simulink model "speed_modelo_definitivo"  (R2022b)
settings: Solver=VariableStepAuto  StartTime=0.0  StopTime=6  FixedStep=0.01  MaxStep=0.00005  RelTol=1e-3
undefined symbols (not defined in the file or in its folder): airgap_drag, corriente_inductancia, Force_drag, frecuencia, frecuencia_freno, FuerzaX_acel, FuerzaX_freno, FuerzaY_acel, Ipeak, mass, p1, p2, pole_length, r, slip, valores_inductancia, VDC, vel_drag, vel_motor_freno
libraries: slpidlib x2
settings Model: Creator=mique  LastModifiedBy=mique
settings SolverCC: ZeroCrossAlgorithm=Adaptive
settings DebuggingCC: IgnoredZcDiagnostic=none

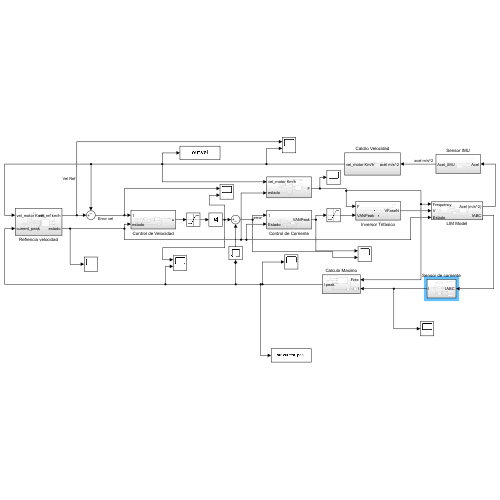
[thumbnail: Simulink's stored preview of the top-level diagram]
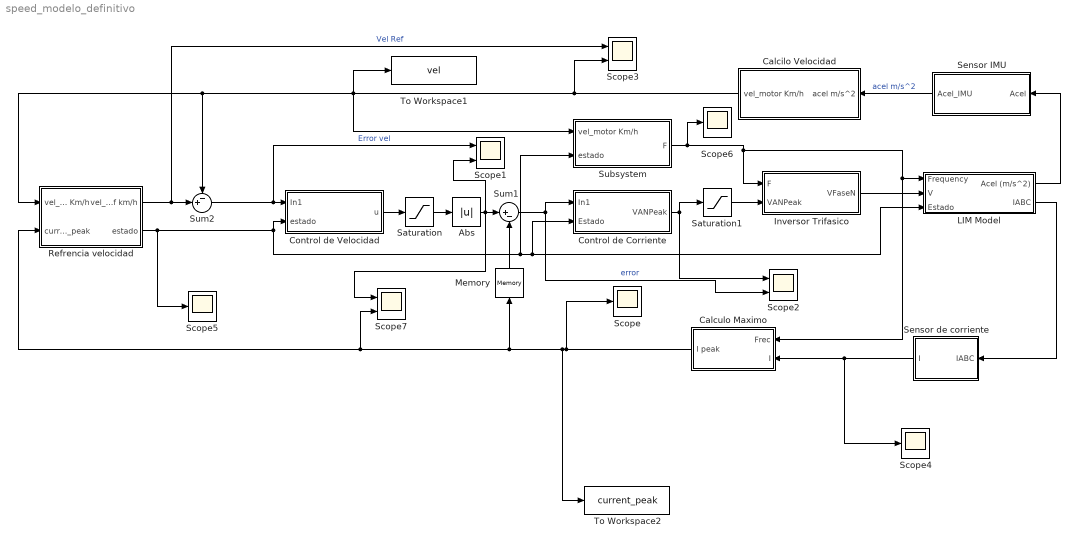
== system speed_modelo_definitivo ==
  Abs : Abs  SaturateOnIntegerOverflow=off
  Calcilo Velocidad : Subsystem
  Calculo Maximo : Subsystem
  Control de Corriente : Subsystem
  Control de Velocidad : Subsystem
  Inversor Trifasico : Subsystem
  LIM Model : Subsystem
  Memory : Memory
  Refrencia velocidad : Subsystem
  Saturation : Saturate  UpperLimit=100  LowerLimit=-100
  Saturation1 : Saturate  UpperLimit=200/sqrt(3)  LowerLimit=0
  Scope{,4..6} (4 alike) : Scope
  Scope{1..3,7} (4 alike) : Scope  NumInputPorts=2
  Sensor IMU : Subsystem
  Sensor de corriente : Subsystem
  Subsystem : Subsystem
  Sum1 : Sum  Inputs=|+-
  Sum2 : Sum  Inputs=-+|
  To Workspace1 : ToWorkspace  VariableName=vel  SampleTime=-1
  To Workspace2 : ToWorkspace  VariableName=current_peak  SaveFormat=Timeseries  SampleTime=-1
  wires:
  LIM Model/1(Acel (m/s^2)) -> Sensor IMU/1(Acel)
  Sum1/1 -> Control de Corriente/1(In1), Scope2/2  "error"
  Refrencia velocidad/1(vel_ref km/h) -> Scope3/1, Sum2/2  "Vel Ref"
  Control de Velocidad/1(u) -> Saturation/1
  Inversor Trifasico/1(VFaseN) -> LIM Model/2("V ")
  Memory/1 -> Sum1/2
  Sensor de corriente/1(I) -> Scope4/1, Calculo Maximo/2(I)
  Control de Corriente/1(VANPeak) -> Saturation1/1, Scope2/1
  Saturation1/1 -> Inversor Trifasico/2(VANPeak)
  Subsystem/1(F) -> Scope6/1, Calculo Maximo/1(Frec), LIM Model/1(Frequency), Inversor Trifasico/1(F)
  Calculo Maximo/1(I peak) -> To Workspace2/1, Scope7/2, Refrencia velocidad/2(current_peak), Memory/1, Scope/1
  LIM Model/2(IABC) -> Sensor de corriente/1(IABC)
  Calcilo Velocidad/1(vel_motor Km/h) -> Scope3/2, Refrencia velocidad/1(vel_motor Km/h), Sum2/1, To Workspace1/1, Subsystem/1(vel_motor Km/h)
  Sensor IMU/1(Acel_IMU) -> Calcilo Velocidad/1(acel m/s^2)  "acel m/s^2"
  Sum2/1 -> Scope1/1, Control de Velocidad/1(In1)  "Error vel"
  Refrencia velocidad/2(estado) -> Scope5/1, Control de Velocidad/2(estado), LIM Model/3(Estado), Control de Corriente/2(Estado), Subsystem/2(estado)
  Saturation/1 -> Abs/1
  Abs/1 -> Scope7/1, Sum1/1, Scope1/2

== system speed_modelo_definitivo/Calcilo Velocidad ==
  acel m/s^2 : Inport
  Gain : Gain  Gain=3.6
  Integrator1 : Integrator
  vel_motor Km/h : Outport
  wires:
  Gain/1 -> vel_motor Km/h/1  "vel_motor Km/h"
  Integrator1/1 -> Gain/1  "vel_motor m/s"
  acel m/s^2/1 -> Integrator1/1

== system speed_modelo_definitivo/Calculo Maximo ==
  Frec : Inport
  I : Inport  Port=2
  Abs : Abs  SaturateOnIntegerOverflow=off
  Clock : Clock
  MATLAB Function : MATLAB Function  TreatAsAtomicUnit=on
  Scope : Scope  NumInputPorts=2
  I peak : Outport
  wires:
  Frec/1 -> MATLAB Function/1(frecuencia)
  I/1 -> MATLAB Function/2(valores), Abs/1
  MATLAB Function/1(maximo) -> I peak/1, Scope/1
  Clock/1 -> MATLAB Function/3(tiempo)
  Abs/1 -> Scope/2

== system speed_modelo_definitivo/Control de Corriente ==
  note: Parametros obtenidos con el PID tuner
  In1 : Inport
  Estado : Inport  Port=2
  Discrete PID Controller1 : slpidlib/PID Controller  Controller=PI  Form=Parallel  TimeDomain=Discrete-time  UseExternalTs=off  SampleTime=0.0002  IntegratorMethod=Forward Euler  FilterMethod=Forward Euler  ControllerParametersSource=internal  P=1  I=25  UseKiTs=off  D=0.3  N=2  UseFilter=on  TunerSelectOption=Transfer Function Based (PID Tuner App)  InitialConditionSource=internal  InitialConditionForIntegrator=0  InitialConditionForFilter=0  DifferentiatorICPrevScaledInput=0  ExternalReset=level  TrackingMode=off  Kt=1  LimitOutput=off  SatLimitsSource=internal  UpperSaturationLimit=VDC/sqrt(3)  LowerSaturationLimit=-VDC/sqrt(3)  LinearizeAsGain=off  AntiWindupMode=back-calculation  Kb=20  LimitIntegrator=off  UpperIntegratorSaturationLimit=15  LowerIntegratorSaturationLimit=-15  POutMin=[]  POutMax=[]  IOutMin=[]  IOutMax=[]  DOutMin=[]  DOutMax=[]  NOutMin=[]  NOutMax=[]  SumOutMin=[]  SumOutMax=[]  SaturationOutMin=[]  SaturationOutMax=[]  PParamMin=[]  PParamMax=[]  IParamMin=[]  IParamMax=[]  DParamMin=[]  DParamMax=[]  NParamMin=[]  NParamMax=[]  KbParamMin=[]  KbParamMax=[]  KtParamMin=[]  KtParamMax=[]  KbOutMin=[]  KbOutMax=[]  KtOutMin=[]  KtOutMax=[]  IntegratorOutMin=[]  IntegratorOutMax=[]  FilterOutMin=[]  FilterOutMax=[]  SumI1OutMin=[]  SumI1OutMax=[]  SumI2OutMin=[]  SumI2OutMax=[]  SumI3OutMin=[]  SumI3OutMax=[]  SumI4OutMin=[]  SumI4OutMax=[]  SumDOutMin=[]  SumDOutMax=[]  DifferentiatorOutMin=[]  DifferentiatorOutMax=[]  FilterDiffOutCoefMin=[]  FilterDiffOutCoefMax=[]  ReciprocalOutMin=[]  ReciprocalOutMax=[]  SumDenOutMin=[]  SumDenOutMax=[]  SumNumOutMin=[]  SumNumOutMax=[]  DivideOutMin=[]  DivideOutMax=[]  UdiffTsProdOutMin=[]  UdiffTsProdOutMax=[]  NTsProdOutMin=[]  NTsProdOutMax=[]  UintegralTsProdOutMin=[]  UintegralTsProdOutMax=[]  UngainTsProdOutMin=[]  UngainTsProdOutMax=[]  ClampingZeroOutDataTypeStr=Inherit: Inherit via back propagation  ClampingZeroOutMin=[]  ClampingZeroOutMax=[]  FilterDenConstantOutDataTypeStr=Inherit: Inherit via back propagation  FilterDenConstantOutMin=[]  FilterDenConstantOutMax=[]  PCopyOutDataTypeStr=Inherit: Inherit via back propagation  PCopyOutMin=[]  PCopyOutMax=[]  NCopyOutDataTypeStr=Inherit: Inherit via back propagation  NCopyOutMin=[]  NCopyOutMax=[]  IntegratorContinuousStateAttributes=''  IntegratorStateMustResolveToSignalObject=off  IntegratorRTWStateStorageClass=Auto  FilterContinuousStateAttributes=''  FilterStateMustResolveToSignalObject=off  FilterRTWStateStorageClass=Auto  ParallelPVariant=InternalParameters  IdealPVariant=Disabled  IVariant=InternalParameters  DVariant=Disabled  IntegratorVariant=Discrete  SatVariant=Disabled  AWVariant=Passthrough  PCopyVariant=Disabled  TRVariant=Disabled  FdbkBlocksVariant=Forward  IdealPFdbkVariant=Disabled  SatFdbkVariant=Disabled  DerivativeFilterVariant=Disabled  NVariant=Disabled  NCopyVariant=Disabled_SignalSpec  FilterICVariant=Disabled  IntegratorICVariant=InternalICs  ExternalResetVariant=ExternalReset  TRSumVariant=Passthrough  SumFdbkVariant=Disabled  SumVariant=Sum_PI  TsampFilterVariant=InternalTs  TsampNgainVariant=Passthrough  TsampIntegralVariant=Passthrough  ExternalSaturationOutDataTypeStr=Inherit: Same as second input
      settings: LibrarySourceBlock=simulink/Discrete/Discrete PID Controller
  MATLAB Function : MATLAB Function  TreatAsAtomicUnit=on
  Memory : Memory
  VANPeak : Outport
  wires:
  In1/1 -> Discrete PID Controller1/1
  Discrete PID Controller1/1 -> MATLAB Function/1(u)
  Estado/1 -> MATLAB Function/2(estado)
  MATLAB Function/1(y) -> VANPeak/1
  MATLAB Function/2(reset) -> Memory/1
  Memory/1 -> Discrete PID Controller1/2

== system speed_modelo_definitivo/Control de Velocidad ==
  note: Parametros obtenidos con el PID tuner
  In1 : Inport
  estado : Inport  Port=2
  Discrete PID Controller1 : slpidlib/PID Controller  Controller=PI  Form=Parallel  TimeDomain=Discrete-time  UseExternalTs=off  SampleTime=0.001  IntegratorMethod=Forward Euler  FilterMethod=Forward Euler  ControllerParametersSource=internal  P=40  I=2  UseKiTs=off  D=0.2  N=10  UseFilter=on  TunerSelectOption=Transfer Function Based (PID Tuner App)  InitialConditionSource=internal  InitialConditionForIntegrator=0  InitialConditionForFilter=0  DifferentiatorICPrevScaledInput=0  ExternalReset=level  TrackingMode=off  Kt=1  LimitOutput=off  SatLimitsSource=internal  UpperSaturationLimit=100  LowerSaturationLimit=-100  LinearizeAsGain=off  AntiWindupMode=clamping  Kb=0.1  LimitIntegrator=off  UpperIntegratorSaturationLimit=15  LowerIntegratorSaturationLimit=-15  POutMin=[]  POutMax=[]  IOutMin=[]  IOutMax=[]  DOutMin=[]  DOutMax=[]  NOutMin=[]  NOutMax=[]  SumOutMin=[]  SumOutMax=[]  SaturationOutMin=[]  SaturationOutMax=[]  PParamMin=[]  PParamMax=[]  IParamMin=[]  IParamMax=[]  DParamMin=[]  DParamMax=[]  NParamMin=[]  NParamMax=[]  KbParamMin=[]  KbParamMax=[]  KtParamMin=[]  KtParamMax=[]  KbOutMin=[]  KbOutMax=[]  KtOutMin=[]  KtOutMax=[]  IntegratorOutMin=[]  IntegratorOutMax=[]  FilterOutMin=[]  FilterOutMax=[]  SumI1OutMin=[]  SumI1OutMax=[]  SumI2OutMin=[]  SumI2OutMax=[]  SumI3OutMin=[]  SumI3OutMax=[]  SumI4OutMin=[]  SumI4OutMax=[]  SumDOutMin=[]  SumDOutMax=[]  DifferentiatorOutMin=[]  DifferentiatorOutMax=[]  FilterDiffOutCoefMin=[]  FilterDiffOutCoefMax=[]  ReciprocalOutMin=[]  ReciprocalOutMax=[]  SumDenOutMin=[]  SumDenOutMax=[]  SumNumOutMin=[]  SumNumOutMax=[]  DivideOutMin=[]  DivideOutMax=[]  UdiffTsProdOutMin=[]  UdiffTsProdOutMax=[]  NTsProdOutMin=[]  NTsProdOutMax=[]  UintegralTsProdOutMin=[]  UintegralTsProdOutMax=[]  UngainTsProdOutMin=[]  UngainTsProdOutMax=[]  ClampingZeroOutDataTypeStr=Inherit: Inherit via back propagation  ClampingZeroOutMin=[]  ClampingZeroOutMax=[]  FilterDenConstantOutDataTypeStr=Inherit: Inherit via back propagation  FilterDenConstantOutMin=[]  FilterDenConstantOutMax=[]  PCopyOutDataTypeStr=Inherit: Inherit via back propagation  PCopyOutMin=[]  PCopyOutMax=[]  NCopyOutDataTypeStr=Inherit: Inherit via back propagation  NCopyOutMin=[]  NCopyOutMax=[]  IntegratorContinuousStateAttributes=''  IntegratorStateMustResolveToSignalObject=off  IntegratorRTWStateStorageClass=Auto  FilterContinuousStateAttributes=''  FilterStateMustResolveToSignalObject=off  FilterRTWStateStorageClass=Auto  ParallelPVariant=InternalParameters  IdealPVariant=Disabled  IVariant=InternalParameters  DVariant=Disabled  IntegratorVariant=Discrete  SatVariant=Disabled  AWVariant=Passthrough  PCopyVariant=Disabled  TRVariant=Disabled  FdbkBlocksVariant=Forward  IdealPFdbkVariant=Disabled  SatFdbkVariant=Disabled  DerivativeFilterVariant=Disabled  NVariant=Disabled  NCopyVariant=Disabled_SignalSpec  FilterICVariant=Disabled  IntegratorICVariant=InternalICs  ExternalResetVariant=ExternalReset  TRSumVariant=Passthrough  SumFdbkVariant=Disabled  SumVariant=Sum_PI  TsampFilterVariant=InternalTs  TsampNgainVariant=Passthrough  TsampIntegralVariant=Passthrough  ExternalSaturationOutDataTypeStr=Inherit: Same as second input
      settings: LibrarySourceBlock=simulink/Discrete/Discrete PID Controller
  MATLAB Function : MATLAB Function  TreatAsAtomicUnit=on
  Memory : Memory
  u : Outport
  wires:
  Discrete PID Controller1/1 -> MATLAB Function/1(i)
  In1/1 -> Discrete PID Controller1/1
  MATLAB Function/1(i_ref) -> u/1
  estado/1 -> MATLAB Function/2(estado)
  MATLAB Function/2(reset) -> Memory/1
  Memory/1 -> Discrete PID Controller1/2

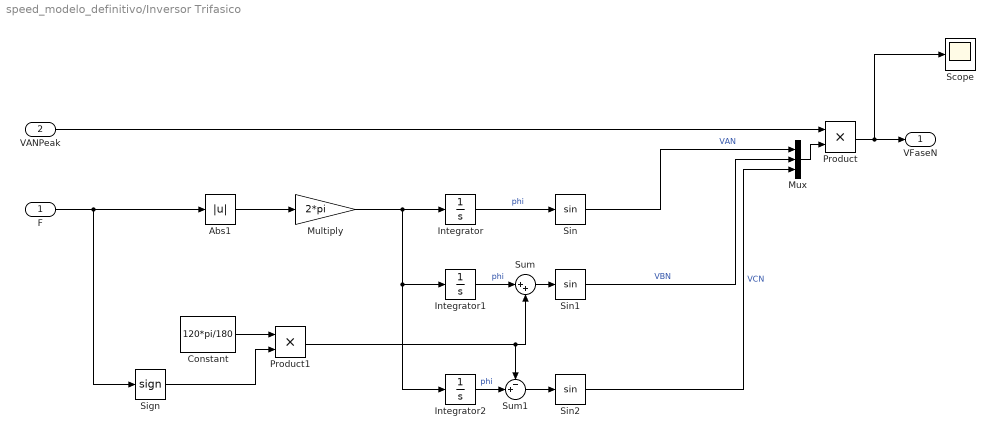
== system speed_modelo_definitivo/Inversor Trifasico ==
  F : Inport
  VANPeak : Inport  Port=2
  Abs1 : Abs  SaturateOnIntegerOverflow=off
  Constant : Constant  Value=120*pi/180
  Integrator : Integrator  WrapState=on  WrappedStateUpperValue=2*pi  WrappedStateLowerValue=0
  Integrator1 : Integrator  WrapState=on  WrappedStateUpperValue=2*pi  WrappedStateLowerValue=0
  Integrator2 : Integrator  WrapState=on  WrappedStateUpperValue=2*pi  WrappedStateLowerValue=0
  Multiply : Gain  Gain=2*pi
  Mux : Mux  Inputs=3
  Product : Product
  Product1 : Product
  Scope : Scope
  Sign : Signum
  Sin : Trigonometry
  Sin1 : Trigonometry
  Sin2 : Trigonometry
  Sum : Sum  Inputs=|++
  Sum1 : Sum  Inputs=-+|
  VFaseN : Outport
  wires:
  Integrator/1 -> Sin/1  "phi"
  Multiply/1 -> Integrator2/1, Integrator1/1, Integrator/1
  VANPeak/1 -> Product/1
  Sin/1 -> Mux/1  "VAN"
  Sin1/1 -> Mux/2  "VBN"
  Sin2/1 -> Mux/3  "VCN"
  Integrator1/1 -> Sum/1  "phi"
  Sum/1 -> Sin1/1
  Sum1/1 -> Sin2/1
  Integrator2/1 -> Sum1/2  "phi"
  Mux/1 -> Product/2
  Product/1 -> Scope/1, VFaseN/1
  F/1 -> Sign/1, Abs1/1
  Abs1/1 -> Multiply/1
  Constant/1 -> Product1/1
  Sign/1 -> Product1/2
  Product1/1 -> Sum1/1, Sum/2

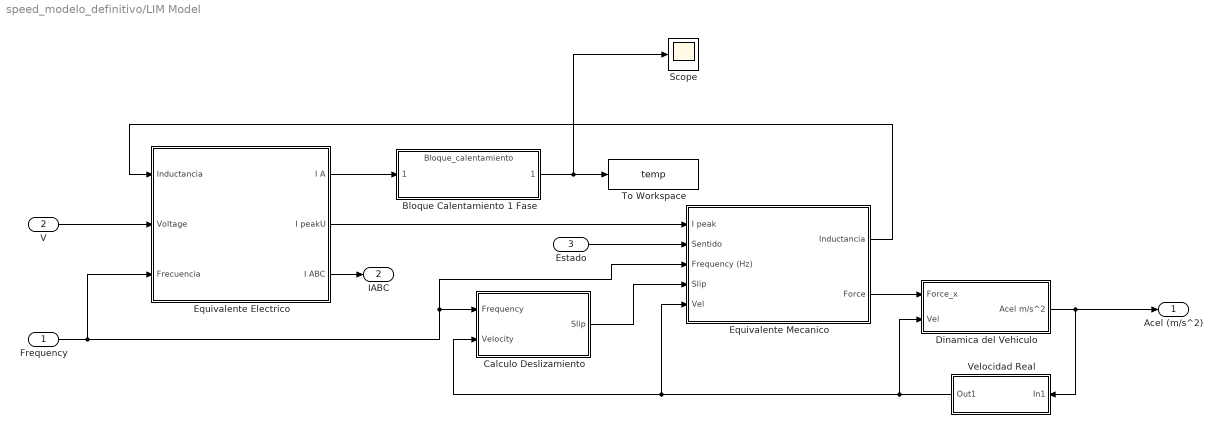
== system speed_modelo_definitivo/LIM Model ==
  Frequency : Inport
  "V " : Inport  Port=2
  Estado : Inport  Port=3
  Bloque Calentamiento 1 Fase : ModelReference  ModelNameDialog=Bloque_calentamiento.slx  SimulationMode=Normal  ModelReferenceVersion=3.9
  Calculo Deslizamiento : Subsystem
  Dinamica del Vehiculo : Subsystem
  Equivalente Electrico : Subsystem
  Equivalente Mecanico : Subsystem
  Scope : Scope
  To Workspace : ToWorkspace  VariableName=temp  SaveFormat=Timeseries  SampleTime=-1
  Velocidad Real : Subsystem
  Acel (m/s^2) : Outport
  IABC : Outport  Port=2
  wires:
  Dinamica del Vehiculo/1(Acel m/s^2) -> Acel (m/s^2)/1, Velocidad Real/1(In1)
  Equivalente Electrico/2(I peakU) -> Equivalente Mecanico/1(I peak)
  Frequency/1 -> Equivalente Electrico/3(Frecuencia), Equivalente Mecanico/3(Frequency (Hz)), Calculo Deslizamiento/1(Frequency)
  "V "/1 -> Equivalente Electrico/2(Voltage)
  Equivalente Electrico/1(I A) -> Bloque Calentamiento 1 Fase/1
  Estado/1 -> Equivalente Mecanico/2(Sentido)
  Calculo Deslizamiento/1(Slip) -> Equivalente Mecanico/4(Slip)
  Equivalente Mecanico/2(Force) -> Dinamica del Vehiculo/1(Force_x)
  Equivalente Electrico/3(I ABC) -> IABC/1
  Velocidad Real/1(Out1) -> Dinamica del Vehiculo/2(Vel), Calculo Deslizamiento/2(Velocity), Equivalente Mecanico/5(Vel)
  Bloque Calentamiento 1 Fase/1 -> Scope/1, To Workspace/1
  Equivalente Mecanico/1(Inductancia) -> Equivalente Electrico/1(Inductancia)

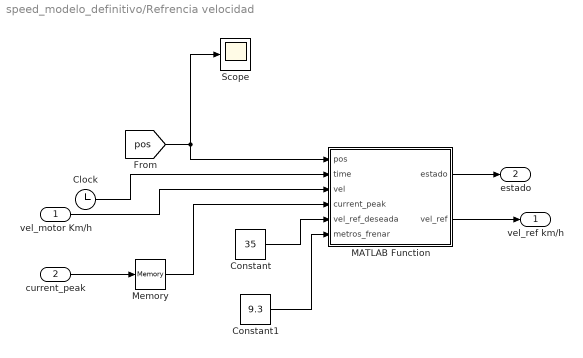
== system speed_modelo_definitivo/Refrencia velocidad ==
  vel_motor Km/h : Inport
  current_peak : Inport  Port=2
  Clock : Clock
  Constant : Constant  Value=35
  Constant1 : Constant  Value=9.3
  MATLAB Function : MATLAB Function  TreatAsAtomicUnit=on
  Memory : Memory
  Scope : Scope
  vel_ref km/h : Outport
  estado : Outport  Port=2
  wires:
  MATLAB Function/2(vel_ref) -> vel_ref km/h/1
  vel_motor Km/h/1 -> MATLAB Function/3(vel)
  Clock/1 -> MATLAB Function/2(time)
  [pos] -> MATLAB Function/1(pos), Scope/1
  current_peak/1 -> Memory/1
  Memory/1 -> MATLAB Function/4(current_peak)
  MATLAB Function/1(estado) -> estado/1
  Constant/1 -> MATLAB Function/5(vel_ref_deseada)
  Constant1/1 -> MATLAB Function/6(metros_frenar)

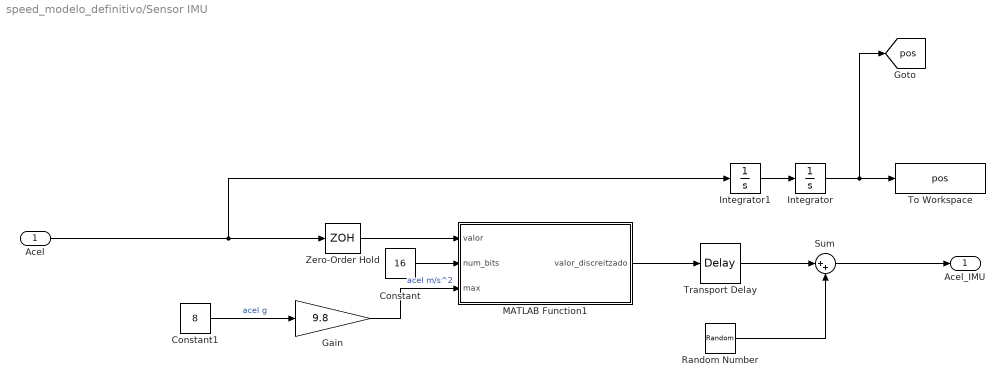
== system speed_modelo_definitivo/Sensor IMU ==
  Acel : Inport
  Constant : Constant  Value=16
  Constant1 : Constant  Value=8
  Gain : Gain  Gain=9.8
  Integrator : Integrator
  Integrator1 : Integrator
  MATLAB Function1 : MATLAB Function  TreatAsAtomicUnit=on
  Random Number : RandomNumber  Variance=0.1  SampleTime=0.001
  Sum : Sum  Inputs=|++
  To Workspace : ToWorkspace  VariableName=pos  SampleTime=-1
  Transport Delay : TransportDelay  DelayTime=0.001
  Zero-Order Hold : ZeroOrderHold  SampleTime=0.001
  Acel_IMU : Outport
  tag scope: pos=global
  wires:
  MATLAB Function1/1(valor_discreitzado) -> Transport Delay/1
  Zero-Order Hold/1 -> MATLAB Function1/1(valor)
  Constant1/1 -> Gain/1  "acel g"
  Constant/1 -> MATLAB Function1/2(num_bits)
  Gain/1 -> MATLAB Function1/3(max)  "acel m/s^2"
  Transport Delay/1 -> Sum/1
  Acel/1 -> Integrator1/1, Zero-Order Hold/1
  Sum/1 -> Acel_IMU/1
  Random Number/1 -> Sum/2
  Integrator/1 -> [pos], To Workspace/1
  Integrator1/1 -> Integrator/1

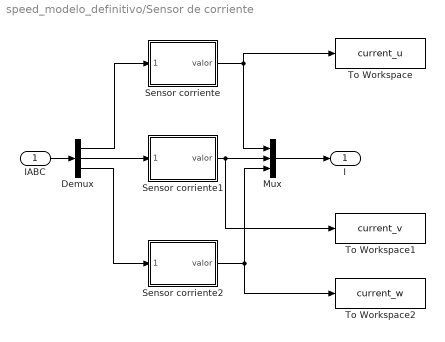
== system speed_modelo_definitivo/Sensor de corriente ==
  IABC : Inport
  Demux : Demux  Outputs=3
  Mux : Mux  Inputs=3
  Sensor corriente : Subsystem
  Sensor corriente1 : Subsystem
  Sensor corriente2 : Subsystem
  To Workspace : ToWorkspace  VariableName=current_u  SaveFormat=Timeseries  SampleTime=-1
  To Workspace1 : ToWorkspace  VariableName=current_v  SaveFormat=Timeseries  SampleTime=-1
  To Workspace2 : ToWorkspace  VariableName=current_w  SaveFormat=Timeseries  SampleTime=-1
  I : Outport
  wires:
  IABC/1 -> Demux/1
  Demux/2 -> Sensor corriente1/1(Current)
  Demux/1 -> Sensor corriente/1(Current)
  Demux/3 -> Sensor corriente2/1(Current)
  Sensor corriente1/1(valor) -> To Workspace1/1, Mux/2
  Mux/1 -> I/1
  Sensor corriente2/1(valor) -> Mux/3, To Workspace2/1
  Sensor corriente/1(valor) -> To Workspace/1, Mux/1

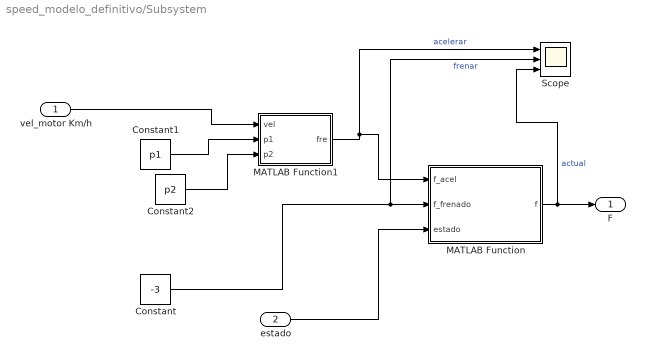
== system speed_modelo_definitivo/Subsystem ==
  vel_motor Km/h : Inport
  estado : Inport  Port=2
  Constant : Constant  Value=-3
  Constant1 : Constant  Value=p1
  Constant2 : Constant  Value=p2
  MATLAB Function : MATLAB Function  TreatAsAtomicUnit=on
  MATLAB Function1 : MATLAB Function  TreatAsAtomicUnit=on
  Scope : Scope  NumInputPorts=3
  F : Outport
  wires:
  vel_motor Km/h/1 -> MATLAB Function1/1(vel)
  estado/1 -> MATLAB Function/3(estado)
  MATLAB Function1/1(fre) -> Scope/1, MATLAB Function/1(f_acel)  "acelerar"
  MATLAB Function/1(f) -> Scope/3, F/1  "actual"
  Constant1/1 -> MATLAB Function1/2(p1)
  Constant2/1 -> MATLAB Function1/3(p2)
  Constant/1 -> Scope/2, MATLAB Function/2(f_frenado)  "frenar"

== system speed_modelo_definitivo/LIM Model/Calculo Deslizamiento ==
  Frequency : Inport
  Velocity : Inport  Port=2
  Constant : Constant  Value=pole_length
  Divide : Product  Inputs=**
  Gain : Gain  Gain=7.2
  MATLAB Function : MATLAB Function  TreatAsAtomicUnit=on
  Slip : Outport
  wires:
  Frequency/1 -> Gain/1
  MATLAB Function/1(slip) -> Slip/1
  Gain/1 -> Divide/2
  Constant/1 -> Divide/1
  Divide/1 -> MATLAB Function/1(we)
  Velocity/1 -> MATLAB Function/2(wm)

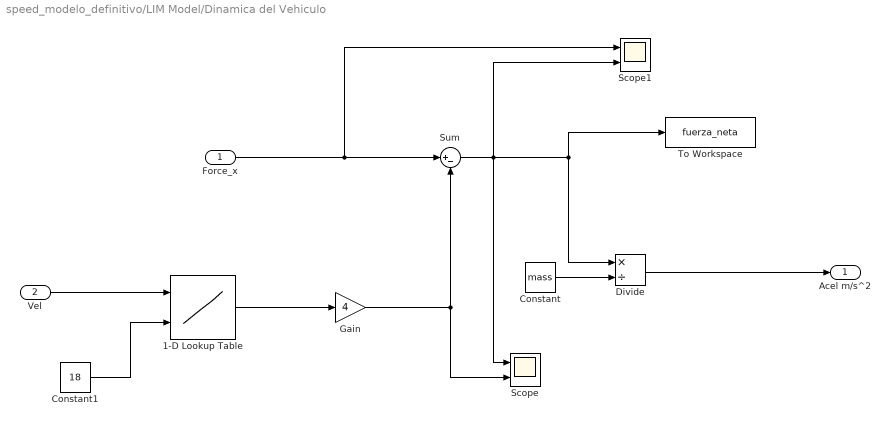
== system speed_modelo_definitivo/LIM Model/Dinamica del Vehiculo ==
  Force_x : Inport
  Vel : Inport  Port=2
  1-D Lookup Table : Lookup_n-D  BreakpointsForDimension1=vel_drag  BreakpointsForDimension2=airgap_drag  Table=Force_drag  InternalRulePriority=Speed  RndMeth=Simplest
      settings: InputPortMap=u0,u1
  Constant : Constant  Value=mass
  Constant1 : Constant  Value=18
  Divide : Product  Inputs=*/
  Gain : Gain  Gain=4
  Scope : Scope  NumInputPorts=2
  Scope1 : Scope  NumInputPorts=2
  Sum : Sum  Inputs=|+-
  To Workspace : ToWorkspace  VariableName=fuerza_neta  SampleTime=-1
  Acel m/s^2 : Outport
  wires:
  Divide/1 -> Acel m/s^2/1
  Constant/1 -> Divide/2
  Force_x/1 -> Sum/1, Scope1/1
  Sum/1 -> To Workspace/1, Divide/1, Scope1/2, Scope/1
  Constant1/1 -> 1-D Lookup Table/2
  1-D Lookup Table/1 -> Gain/1
  Gain/1 -> Scope/2, Sum/2
  Vel/1 -> 1-D Lookup Table/1

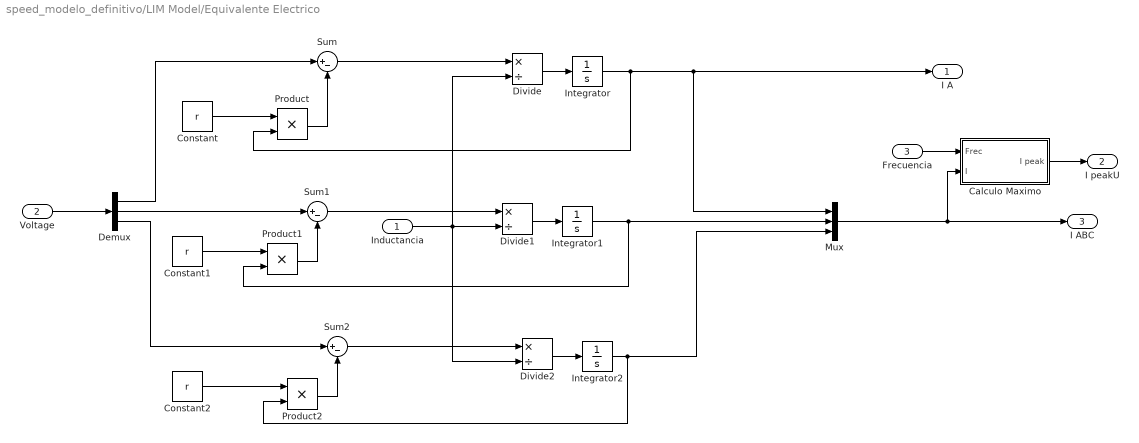
== system speed_modelo_definitivo/LIM Model/Equivalente Electrico ==
  Inductancia : Inport
  Voltage : Inport  Port=2
  Frecuencia : Inport  Port=3
  Calculo Maximo : Subsystem
  Constant : Constant  Value=r
  Constant1 : Constant  Value=r
  Constant2 : Constant  Value=r
  Demux : Demux  Outputs=3
  Divide : Product  Inputs=*/
  Divide1 : Product  Inputs=*/
  Divide2 : Product  Inputs=*/
  Integrator : Integrator
  Integrator1 : Integrator
  Integrator2 : Integrator
  Mux : Mux  Inputs=3
  Product : Product
  Product1 : Product
  Product2 : Product
  Sum : Sum  Inputs=|+-
  Sum1 : Sum  Inputs=|+-
  Sum2 : Sum  Inputs=|+-
  I A : Outport
  I peakU : Outport  Port=2
  I ABC : Outport  Port=3
  wires:
  Integrator/1 -> I A/1, Mux/1, Product/2
  Constant/1 -> Product/1
  Product/1 -> Sum/2
  Divide/1 -> Integrator/1
  Sum/1 -> Divide/1
  Sum1/1 -> Divide1/1
  Product1/1 -> Sum1/2
  Divide1/1 -> Integrator1/1
  Integrator1/1 -> Mux/2, Product1/2
  Constant1/1 -> Product1/1
  Integrator2/1 -> Mux/3, Product2/2
  Constant2/1 -> Product2/1
  Sum2/1 -> Divide2/1
  Divide2/1 -> Integrator2/1
  Product2/1 -> Sum2/2
  Voltage/1 -> Demux/1
  Demux/1 -> Sum/1
  Demux/2 -> Sum1/1
  Demux/3 -> Sum2/1
  Mux/1 -> Calculo Maximo/2(I), I ABC/1
  Frecuencia/1 -> Calculo Maximo/1(Frec)
  Calculo Maximo/1(I peak) -> I peakU/1
  Inductancia/1 -> Divide2/2, Divide1/2, Divide/2

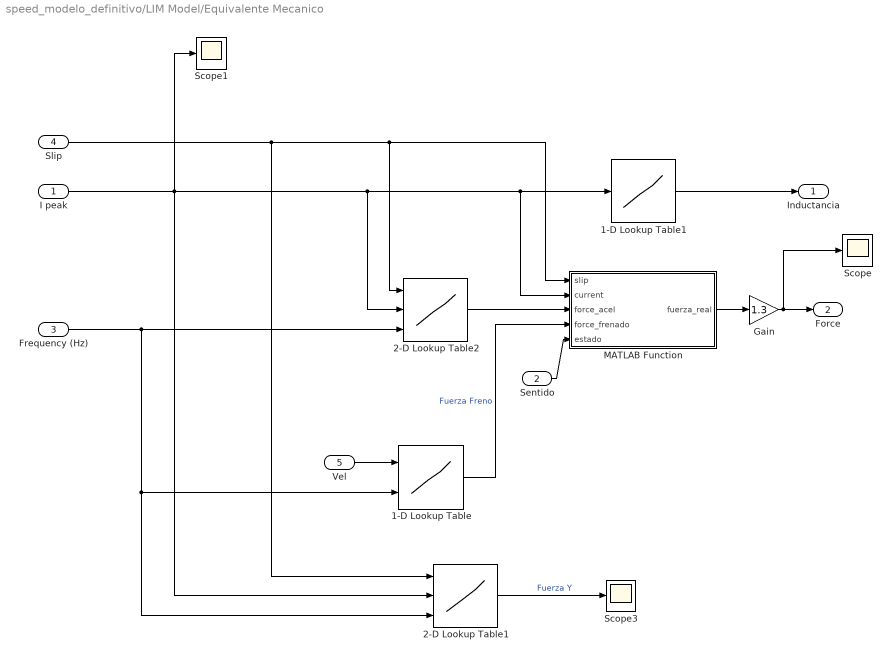
== system speed_modelo_definitivo/LIM Model/Equivalente Mecanico ==
  I peak : Inport
  Sentido : Inport  Port=2
  Frequency (Hz) : Inport  Port=3
  Slip : Inport  Port=4
  Vel : Inport  Port=5
  1-D Lookup Table : Lookup_n-D  BreakpointsForDimension1=vel_motor_freno  BreakpointsForDimension2=frecuencia_freno  Table=FuerzaX_freno  InternalRulePriority=Speed  RndMeth=Simplest
      settings: InputPortMap=u0,u1
  1-D Lookup Table1 : Lookup_n-D  NumberOfTableDimensions=1  BreakpointsForDimension1=corriente_inductancia  Table=valores_inductancia  InternalRulePriority=Speed  RndMeth=Simplest
  2-D Lookup Table1 : Lookup_n-D  NumberOfTableDimensions=3  BreakpointsForDimension1=slip  BreakpointsForDimension2=Ipeak  BreakpointsForDimension3=frecuencia  Table=FuerzaY_acel  InterpMethod=Nearest  InternalRulePriority=Speed  RndMeth=Simplest
      settings: InputPortMap=u0,u1,u2
  2-D Lookup Table2 : Lookup_n-D  NumberOfTableDimensions=3  BreakpointsForDimension1=slip  BreakpointsForDimension2=Ipeak  BreakpointsForDimension3=frecuencia  Table=FuerzaX_acel  InternalRulePriority=Speed  RndMeth=Simplest
      settings: InputPortMap=u0,u1,u2
  Gain : Gain  Gain=1.3
  MATLAB Function : MATLAB Function  TreatAsAtomicUnit=on
  Scope : Scope
  Scope1 : Scope
  Scope3 : Scope
  Inductancia : Outport
  Force : Outport  Port=2
  wires:
  Frequency (Hz)/1 -> 2-D Lookup Table2/3, 1-D Lookup Table/2, 2-D Lookup Table1/3
  I peak/1 -> Scope1/1, 1-D Lookup Table1/1, MATLAB Function/2(current), 2-D Lookup Table2/2, 2-D Lookup Table1/2
  Slip/1 -> 2-D Lookup Table1/1, MATLAB Function/1(slip), 2-D Lookup Table2/1
  2-D Lookup Table2/1 -> MATLAB Function/3(force_acel)
  2-D Lookup Table1/1 -> Scope3/1  "Fuerza Y"
  Sentido/1 -> MATLAB Function/5(estado)
  MATLAB Function/1(fuerza_real) -> Gain/1
  Gain/1 -> Scope/1, Force/1
  Vel/1 -> 1-D Lookup Table/1
  1-D Lookup Table1/1 -> Inductancia/1
  1-D Lookup Table/1 -> MATLAB Function/4(force_frenado)  "Fuerza Freno"

== system speed_modelo_definitivo/LIM Model/Velocidad Real ==
  In1 : Inport
  Gain1 : Gain  Gain=3.6
  Integrator : Integrator
  Out1 : Outport
  wires:
  Integrator/1 -> Gain1/1
  Gain1/1 -> Out1/1
  In1/1 -> Integrator/1

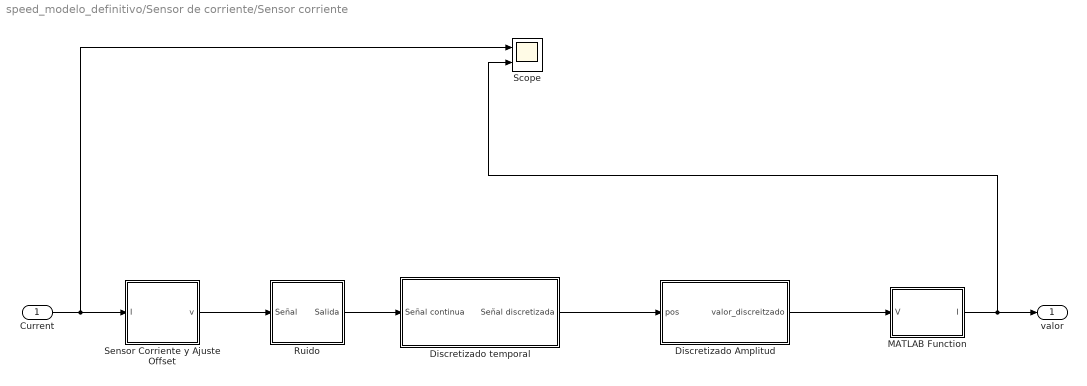
== system speed_modelo_definitivo/Sensor de corriente/Sensor corriente ==
  Current : Inport
  Discretizado Amplitud : Subsystem  mask{Num_Val=4069, Max=4, Min=1}
      mask prompts: Num_Val "Numero de valores distintos"; Max "Maximo valor"; Min "Minimo valor"
  Discretizado temporal : Subsystem  mask{Tiempo_Discretizado=0.0002}
      mask prompts: Tiempo_Discretizado "Tiempo de discretizacion (s)"
      mask DialogControl DescGroupVar Prompt: Discretiza una señal mediante un ZOH con un tiempo definido
  MATLAB Function : MATLAB Function  TreatAsAtomicUnit=on
  Ruido : Subsystem  mask{M=0, V=0.000003, f=5000}
      mask prompts: M "Media"; V "Varianza"; f "Frecuencia (Hz)"
      mask init:
      | T=1/f;
      mask DialogControl DescGroupVar Prompt: Añadidor de Ruido
      mask DialogControl DescTextVar Prompt: Añade un ruido blanco Gausiano con los siguientes valores:
  Scope : Scope  NumInputPorts=2
  Sensor Corriente y Ajuste Offset : Subsystem  mask{offset=0.0001, max=off}
      mask prompts: max "Offset positivo"
      mask init:
      | if(max==true)
      |         offset=abs(offset);
      | 
      |     else
      |         offset=-offset;
      |     end
  valor : Outport
  wires:
  Discretizado Amplitud/1(valor_discreitzado) -> MATLAB Function/1(V)
  Discretizado temporal/1(Señal discretizada) -> Discretizado Amplitud/1(pos)
  Sensor Corriente y Ajuste Offset/1(v) -> Ruido/1(Señal)
  Ruido/1(Salida) -> Discretizado temporal/1(Señal continua)
  Current/1 -> Scope/1, Sensor Corriente y Ajuste Offset/1(I)
  MATLAB Function/1(I) -> Scope/2, valor/1

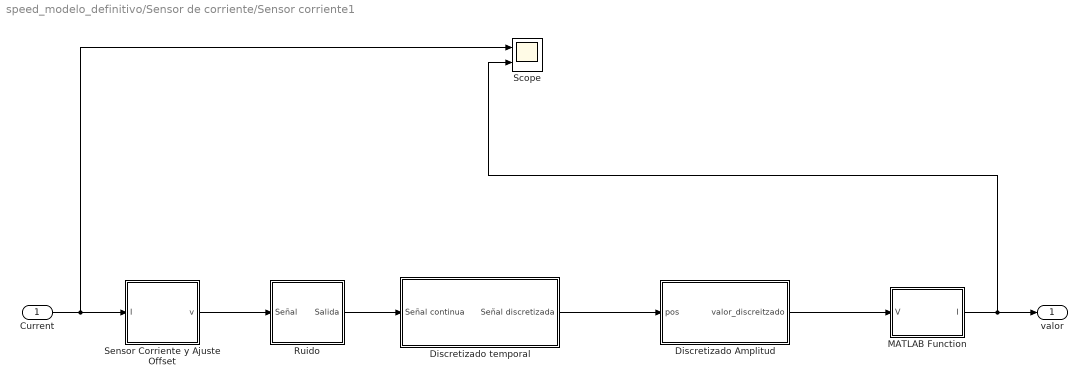
== system speed_modelo_definitivo/Sensor de corriente/Sensor corriente1 ==
  Current : Inport
  Discretizado Amplitud : Subsystem  mask{Num_Val=4069, Max=4, Min=1}
      mask prompts: Num_Val "Numero de valores distintos"; Max "Maximo valor"; Min "Minimo valor"
  Discretizado temporal : Subsystem  mask{Tiempo_Discretizado=0.0002}
      mask prompts: Tiempo_Discretizado "Tiempo de discretizacion (s)"
      mask DialogControl DescGroupVar Prompt: Discretiza una señal mediante un ZOH con un tiempo definido
  MATLAB Function : MATLAB Function  TreatAsAtomicUnit=on
  Ruido : Subsystem  mask{M=0, V=0.000003, f=5000}
      mask prompts: M "Media"; V "Varianza"; f "Frecuencia (Hz)"
      mask init:
      | T=1/f;
      mask DialogControl DescGroupVar Prompt: Añadidor de Ruido
      mask DialogControl DescTextVar Prompt: Añade un ruido blanco Gausiano con los siguientes valores:
  Scope : Scope  NumInputPorts=2
  Sensor Corriente y Ajuste Offset : Subsystem  mask{offset=0.0001, max=off}
      mask prompts: max "Offset positivo"
      mask init:
      | if(max==true)
      |         offset=abs(offset);
      | 
      |     else
      |         offset=-offset;
      |     end
  valor : Outport
  wires:
  MATLAB Function/1(I) -> valor/1, Scope/2
  Current/1 -> Sensor Corriente y Ajuste Offset/1(I), Scope/1
  Ruido/1(Salida) -> Discretizado temporal/1(Señal continua)
  Sensor Corriente y Ajuste Offset/1(v) -> Ruido/1(Señal)
  Discretizado temporal/1(Señal discretizada) -> Discretizado Amplitud/1(pos)
  Discretizado Amplitud/1(valor_discreitzado) -> MATLAB Function/1(V)

== system speed_modelo_definitivo/Sensor de corriente/Sensor corriente2 ==
  Current : Inport
  Discretizado Amplitud : Subsystem  mask{Num_Val=4069, Max=4, Min=1}
      mask prompts: Num_Val "Numero de valores distintos"; Max "Maximo valor"; Min "Minimo valor"
  Discretizado temporal : Subsystem  mask{Tiempo_Discretizado=0.0002}
      mask prompts: Tiempo_Discretizado "Tiempo de discretizacion (s)"
      mask DialogControl DescGroupVar Prompt: Discretiza una señal mediante un ZOH con un tiempo definido
  MATLAB Function : MATLAB Function  TreatAsAtomicUnit=on
  Ruido : Subsystem  mask{M=0, V=0.000003, f=5000}
      mask prompts: M "Media"; V "Varianza"; f "Frecuencia (Hz)"
      mask init:
      | T=1/f;
      mask DialogControl DescGroupVar Prompt: Añadidor de Ruido
      mask DialogControl DescTextVar Prompt: Añade un ruido blanco Gausiano con los siguientes valores:
  Scope : Scope  NumInputPorts=2
  Sensor Corriente y Ajuste Offset : Subsystem  mask{offset=0.0001, max=off}
      mask prompts: max "Offset positivo"
      mask init:
      | if(max==true)
      |         offset=abs(offset);
      | 
      |     else
      |         offset=-offset;
      |     end
  valor : Outport
  wires:
  Discretizado Amplitud/1(valor_discreitzado) -> MATLAB Function/1(V)
  Discretizado temporal/1(Señal discretizada) -> Discretizado Amplitud/1(pos)
  Sensor Corriente y Ajuste Offset/1(v) -> Ruido/1(Señal)
  Ruido/1(Salida) -> Discretizado temporal/1(Señal continua)
  Current/1 -> Scope/1, Sensor Corriente y Ajuste Offset/1(I)
  MATLAB Function/1(I) -> Scope/2, valor/1

== system speed_modelo_definitivo/LIM Model/Equivalente Electrico/Calculo Maximo ==
  Frec : Inport
  I : Inport  Port=2
  Clock : Clock
  MATLAB Function : MATLAB Function  TreatAsAtomicUnit=on
  I peak : Outport
  wires:
  Frec/1 -> MATLAB Function/1(frecuencia)
  I/1 -> MATLAB Function/2(valores)
  MATLAB Function/1(maximo) -> I peak/1
  Clock/1 -> MATLAB Function/3(tiempo)

== system speed_modelo_definitivo/Sensor de corriente/Sensor corriente/Discretizado Amplitud ==
  pos : Inport
  Constant : Constant  Value=Num_Val
  Constant1 : Constant  Value=Max
  Constant2 : Constant  Value=Min
  MATLAB Function1 : MATLAB Function  TreatAsAtomicUnit=on
  valor_discreitzado : Outport
  wires:
  pos/1 -> MATLAB Function1/1(valor)
  Constant2/1 -> MATLAB Function1/4(min)
  Constant/1 -> MATLAB Function1/2(num_valores)
  Constant1/1 -> MATLAB Function1/3(max)
  MATLAB Function1/1(valor_discreitzado) -> valor_discreitzado/1

== system speed_modelo_definitivo/Sensor de corriente/Sensor corriente/Discretizado temporal ==
  Señal continua : Inport
  Zero-Order Hold : ZeroOrderHold  SampleTime=Tiempo_Discretizado
  Señal discretizada : Outport
  wires:
  Zero-Order Hold/1 -> Señal discretizada/1
  Señal continua/1 -> Zero-Order Hold/1

== system speed_modelo_definitivo/Sensor de corriente/Sensor corriente/Ruido ==
  Señal : Inport
  Ruido : RandomNumber  Mean=M  Variance=V  Seed=10  SampleTime=T
  Sum : Sum  Inputs=|++
  Salida : Outport
  wires:
  Sum/1 -> Salida/1
  Ruido/1 -> Sum/1
  Señal/1 -> Sum/2

== system speed_modelo_definitivo/Sensor de corriente/Sensor corriente/Sensor Corriente y Ajuste Offset ==
  I : Inport
  Constant : Constant  Value=offset
  Sensor : MATLAB Function  TreatAsAtomicUnit=on
  v : Outport
  wires:
  I/1 -> Sensor/1(I)
  Constant/1 -> Sensor/2(offset)
  Sensor/1(V_o) -> v/1

== system speed_modelo_definitivo/Sensor de corriente/Sensor corriente1/Discretizado Amplitud ==
  pos : Inport
  Constant : Constant  Value=Num_Val
  Constant1 : Constant  Value=Max
  Constant2 : Constant  Value=Min
  MATLAB Function1 : MATLAB Function  TreatAsAtomicUnit=on
  valor_discreitzado : Outport
  wires:
  MATLAB Function1/1(valor_discreitzado) -> valor_discreitzado/1
  Constant1/1 -> MATLAB Function1/3(max)
  Constant/1 -> MATLAB Function1/2(num_valores)
  Constant2/1 -> MATLAB Function1/4(min)
  pos/1 -> MATLAB Function1/1(valor)

== system speed_modelo_definitivo/Sensor de corriente/Sensor corriente1/Discretizado temporal ==
  Señal continua : Inport
  Zero-Order Hold : ZeroOrderHold  SampleTime=Tiempo_Discretizado
  Señal discretizada : Outport
  wires:
  Señal continua/1 -> Zero-Order Hold/1
  Zero-Order Hold/1 -> Señal discretizada/1

== system speed_modelo_definitivo/Sensor de corriente/Sensor corriente1/Ruido ==
  Señal : Inport
  Ruido : RandomNumber  Mean=M  Variance=V  Seed=10  SampleTime=T
  Sum : Sum  Inputs=|++
  Salida : Outport
  wires:
  Señal/1 -> Sum/2
  Ruido/1 -> Sum/1
  Sum/1 -> Salida/1

== system speed_modelo_definitivo/Sensor de corriente/Sensor corriente1/Sensor Corriente y Ajuste Offset ==
  I : Inport
  Constant : Constant  Value=offset
  Sensor : MATLAB Function  TreatAsAtomicUnit=on
  v : Outport
  wires:
  Sensor/1(V_o) -> v/1
  Constant/1 -> Sensor/2(offset)
  I/1 -> Sensor/1(I)

== system speed_modelo_definitivo/Sensor de corriente/Sensor corriente2/Discretizado Amplitud ==
  pos : Inport
  Constant : Constant  Value=Num_Val
  Constant1 : Constant  Value=Max
  Constant2 : Constant  Value=Min
  MATLAB Function1 : MATLAB Function  TreatAsAtomicUnit=on
  valor_discreitzado : Outport
  wires:
  pos/1 -> MATLAB Function1/1(valor)
  Constant2/1 -> MATLAB Function1/4(min)
  Constant/1 -> MATLAB Function1/2(num_valores)
  Constant1/1 -> MATLAB Function1/3(max)
  MATLAB Function1/1(valor_discreitzado) -> valor_discreitzado/1

== system speed_modelo_definitivo/Sensor de corriente/Sensor corriente2/Discretizado temporal ==
  Señal continua : Inport
  Zero-Order Hold : ZeroOrderHold  SampleTime=Tiempo_Discretizado
  Señal discretizada : Outport
  wires:
  Zero-Order Hold/1 -> Señal discretizada/1
  Señal continua/1 -> Zero-Order Hold/1

== system speed_modelo_definitivo/Sensor de corriente/Sensor corriente2/Ruido ==
  Señal : Inport
  Ruido : RandomNumber  Mean=M  Variance=V  Seed=10  SampleTime=T
  Sum : Sum  Inputs=|++
  Salida : Outport
  wires:
  Sum/1 -> Salida/1
  Ruido/1 -> Sum/1
  Señal/1 -> Sum/2

== system speed_modelo_definitivo/Sensor de corriente/Sensor corriente2/Sensor Corriente y Ajuste Offset ==
  I : Inport
  Constant : Constant  Value=offset
  Sensor : MATLAB Function  TreatAsAtomicUnit=on
  v : Outport
  wires:
  I/1 -> Sensor/1(I)
  Constant/1 -> Sensor/2(offset)
  Sensor/1(V_o) -> v/1

== matlab function speed_modelo_definitivo/Control de Corriente/MATLAB Function ==
  data: u input; y output; estado input; reset output
function [y,reset] = fcn(u, estado)

if estado==3 || estado==0
    y=0;
    reset=1;
else
    y=u;
    reset=0;
end

== matlab function speed_modelo_definitivo/Calculo Maximo/MATLAB Function ==
  settings: updateMethod=DISCRETE
  data: frecuencia input; maximo output; valores input; tiempo input
function maximo = fcn(frecuencia,valores,tiempo)

   persistent antiguo_maximo
    if isempty(antiguo_maximo)
       antiguo_maximo=0;
    end
    persistent t_maximo
    if isempty(t_maximo)
       t_maximo=0;
    end

   persistent posible_nuevo_maximo
    if isempty(posible_nuevo_maximo)
       posible_nuevo_maximo=0;
    end
    persistent posible_t_maximo
    if isempty(posible_t_maximo)
       posible_t_maximo=0;
    end

periodo=1/abs(frecuencia);
valor=max(abs(valores));

if valor>=antiguo_maximo
    maximo=valor;
    antiguo_maximo=valor;
    t_maximo=tiempo;
    posible_nuevo_maximo=0;
    posible_t_maximo=tiempo;

else
    maximo=antiguo_maximo;

    if tiempo>t_maximo+0.1*periodo
        if valor>=posible_nuevo_maximo
            posible_nuevo_maximo=valor;
            posible_t_maximo=tiempo;
        end
    end
    if tiempo>t_maximo+0.6*periodo
        maximo=posible_nuevo_maximo;
        antiguo_maximo=posible_nuevo_maximo;
        posible_nuevo_maximo=0;
        t_maximo=posible_t_maximo;

    end
end

== matlab function speed_modelo_definitivo/Sensor de corriente/Sensor corriente1/MATLAB Function ==
  data: V input; I output
function I = fcn(V)

I=(V-2.5)/0.005;

== matlab function speed_modelo_definitivo/Sensor de corriente/Sensor corriente1/Sensor Corriente y Ajuste Offset/Sensor ==
  data: I input; V_o output; offset input
function V_o = Sensor_L01Z300S05(I,offset)
Vcc=5;
if(I>300)
    I=300;
end
if(I<-300)
    I=-300;
end
V_ref=Vcc/2;
V_o=V_ref+0.005*I;

V_o=V_o+offset;

end

== matlab function speed_modelo_definitivo/LIM Model/Equivalente Mecanico/MATLAB Function ==
  data: slip input; fuerza_real output; current input; force_acel input; force_frenado input; estado input
function fuerza_real = fcn(slip,current,force_acel,force_frenado,estado)

if estado==2
    force=force_frenado;
else
    force=force_acel;
end

if slip == 0 || current<6 && current>-6 || estado==0
    fuerza_real=0;
else
    fuerza_real=force;
end

== matlab function speed_modelo_definitivo/Sensor de corriente/Sensor corriente2/Discretizado Amplitud/MATLAB Function1 ==
  data: valor input; valor_discreitzado output; num_valores input; max input; min input
function valor_discreitzado  = fcn(valor,num_valores,max,min)

if(valor>max)
    valor_discreitzado=max;
    return
end
if(valor<min)
    valor_discreitzado=min;
    return
end


valor_escalon=(max-min)/(num_valores-1);


i=min;
 while(i<max)
    if(i+valor_escalon/2>valor)
        valor_discreitzado=i;
        return
    end
    i=i+valor_escalon;
end



      valor_discreitzado=max;
end

== matlab function speed_modelo_definitivo/Sensor de corriente/Sensor corriente2/MATLAB Function ==
  data: V input; I output
function I = fcn(V)

I=(V-2.5)/0.005;

== matlab function speed_modelo_definitivo/Sensor de corriente/Sensor corriente2/Sensor Corriente y Ajuste Offset/Sensor ==
  data: I input; V_o output; offset input
function V_o = Sensor_L01Z300S05(I,offset)
Vcc=5;
if(I>300)
    I=300;
end
if(I<-300)
    I=-300;
end
V_ref=Vcc/2;
V_o=V_ref+0.005*I;

V_o=V_o+offset;

end

== matlab function speed_modelo_definitivo/Refrencia velocidad/MATLAB Function ==
  settings: updateMethod=DISCRETE
  data: pos input; estado output; time input; vel input; vel_ref output; current_peak input; vel_ref_deseada input; metros_frenar input
function [estado,vel_ref] = fcn(pos,time,vel,current_peak,vel_ref_deseada,metros_frenar)

persistent estado_ant
    if isempty(estado_ant)
       estado_ant=0;
    end


vel_ref=0;
estado=estado_ant;

switch estado_ant
    case 0
        vel_ref=0;
        if time>1 && time<2 %Orden de Arrancar
            estado=1;
            vel_ref=vel_ref_deseada;
        end

    case 1
        vel_ref=vel_ref_deseada;
        if pos>metros_frenar %Final del tubo, empezar a frenar
            estado=3;
        end
    case 2

        if vel<0
            estado=0;
        end
    case 3
        vel_ref=0;
        if current_peak< 5
            estado=2;
        end
end

estado_ant=estado;

== matlab function speed_modelo_definitivo/Control de Velocidad/MATLAB Function ==
  data: i input; i_ref output; estado input; reset output
function [i_ref,reset] = fcn(i,estado)

i_ref=0;

if estado==3 || estado==0
    i_ref=0;
    reset=1;
else
    reset=0;
    if estado==1 && i>0
        i_ref=i;
    end
    if estado==2 && i<0
        i_ref=i;
    end

end

== matlab function speed_modelo_definitivo/Sensor de corriente/Sensor corriente/Discretizado Amplitud/MATLAB Function1 ==
  data: valor input; valor_discreitzado output; num_valores input; max input; min input
function valor_discreitzado  = fcn(valor,num_valores,max,min)

if(valor>max)
    valor_discreitzado=max;
    return
end
if(valor<min)
    valor_discreitzado=min;
    return
end


valor_escalon=(max-min)/(num_valores-1);


i=min;
 while(i<max)
    if(i+valor_escalon/2>valor)
        valor_discreitzado=i;
        return
    end
    i=i+valor_escalon;
end



      valor_discreitzado=max;
end

== matlab function speed_modelo_definitivo/LIM Model/Equivalente Electrico/Calculo Maximo/MATLAB Function ==
  settings: updateMethod=DISCRETE
  data: frecuencia input; maximo output; valores input; tiempo input
function maximo = fcn(frecuencia,valores,tiempo)

   persistent antiguo_maximo
    if isempty(antiguo_maximo)
       antiguo_maximo=0;
    end
    persistent t_maximo
    if isempty(t_maximo)
       t_maximo=0;
    end

   persistent posible_nuevo_maximo
    if isempty(posible_nuevo_maximo)
       posible_nuevo_maximo=0;
    end
    persistent posible_t_maximo
    if isempty(posible_t_maximo)
       posible_t_maximo=0;
    end

periodo=1/abs(frecuencia);
valor=max(abs(valores));

if valor>=antiguo_maximo
    maximo=valor;
    antiguo_maximo=valor;
    t_maximo=tiempo;
    posible_nuevo_maximo=0;
    posible_t_maximo=tiempo;

else
    maximo=antiguo_maximo;

    if tiempo>t_maximo+0.1*periodo
        if valor>=posible_nuevo_maximo
            posible_nuevo_maximo=valor;
            posible_t_maximo=tiempo;
        end
    end
    if tiempo>t_maximo+0.6*periodo
        maximo=posible_nuevo_maximo;
        antiguo_maximo=posible_nuevo_maximo;
        posible_nuevo_maximo=0;
        t_maximo=posible_t_maximo;

    end
end

== matlab function speed_modelo_definitivo/LIM Model/Calculo Deslizamiento/MATLAB Function ==
  data: we input; slip output; wm input
function slip = fcn(we,wm)

slip = (we-wm)/we;

== matlab function speed_modelo_definitivo/Subsystem/MATLAB Function1 ==
  data: vel input; fre output; p1 input; p2 input
function fre = fcn(vel,p1,p2)

fre=p2+p1*vel;

== matlab function speed_modelo_definitivo/Subsystem/MATLAB Function ==
  data: f_acel input; f output; f_frenado input; estado input
function f= fcn(f_acel,f_frenado,estado)

if estado==2
    f=f_frenado;
else
    f=f_acel;
end

== matlab function speed_modelo_definitivo/Sensor de corriente/Sensor corriente1/Discretizado Amplitud/MATLAB Function1 ==
  data: valor input; valor_discreitzado output; num_valores input; max input; min input
function valor_discreitzado  = fcn(valor,num_valores,max,min)

if(valor>max)
    valor_discreitzado=max;
    return
end
if(valor<min)
    valor_discreitzado=min;
    return
end


valor_escalon=(max-min)/(num_valores-1);


i=min;
 while(i<max)
    if(i+valor_escalon/2>valor)
        valor_discreitzado=i;
        return
    end
    i=i+valor_escalon;
end



      valor_discreitzado=max;
end

== matlab function speed_modelo_definitivo/Sensor de corriente/Sensor corriente/MATLAB Function ==
  data: V input; I output
function I = fcn(V)

I=(V-2.5)/0.005;

== matlab function speed_modelo_definitivo/Sensor IMU/MATLAB Function1 ==
  data: valor input; valor_discreitzado output; num_bits input; max input
function valor_discreitzado  = fcn(valor,num_bits,max)

min=-max;
num_valores=2^num_bits;
if(valor>max)
    valor_discreitzado=max;
    return
end
if(valor<min)
    valor_discreitzado=min;
    return
end


valor_escalon=(max-min)/(num_valores-1);


i=min;
 while(i<max)
    if(i+valor_escalon/2>valor)
        valor_discreitzado=i;
        return
    end
    i=i+valor_escalon;
end



      valor_discreitzado=max;
end

== matlab function speed_modelo_definitivo/Sensor de corriente/Sensor corriente/Sensor Corriente y Ajuste Offset/Sensor ==
  data: I input; V_o output; offset input
function V_o = Sensor_L01Z300S05(I,offset)
Vcc=5;
if(I>300)
    I=300;
end
if(I<-300)
    I=-300;
end
V_ref=Vcc/2;
V_o=V_ref+0.005*I;

V_o=V_o+offset;

end
